simulink model "DC_MOTOR_CONTROL_SIMULACION"  (R2022b)
settings: Solver=ode45  StartTime=0.0  StopTime=100  RelTol=1e-3
values from neighbouring files (symbols this model uses):
  B = 5.076    [dc_motor_control_design.m]
libraries: fod x1
settings Model: Creator=mario  LastModifiedBy=mario
settings SolverCC: ZeroCrossAlgorithm=Adaptive
settings DebuggingCC: IgnoredZcDiagnostic=none

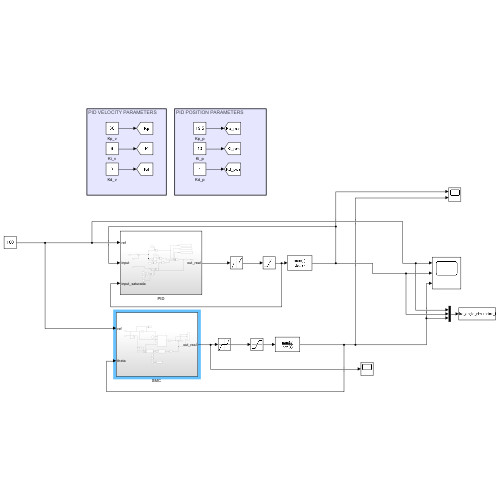
[thumbnail: Simulink's stored preview of the top-level diagram]
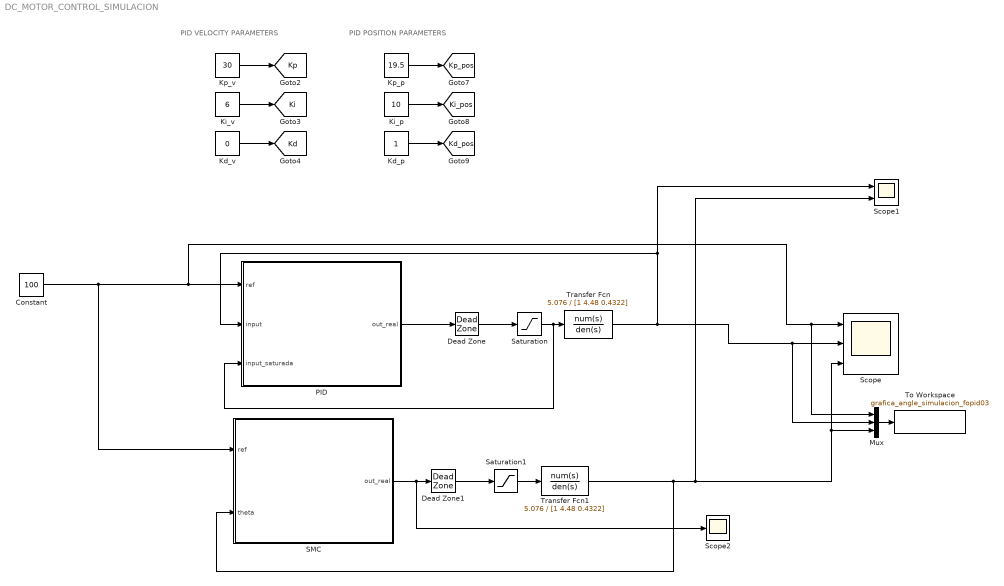
== system DC_MOTOR_CONTROL_SIMULACION ==
  note: PID VELOCITY PARAMETERS
  note: PID POSITION PARAMETERS
  Constant : Constant  Value=100
  Dead Zone : DeadZone  LowerValue=-70  UpperValue=70
  Dead Zone1 : DeadZone  LowerValue=-70  UpperValue=70
  Kd_p : Constant
  Kd_v : Constant  Value=0
  Ki_p : Constant  Value=10
  Ki_v : Constant  Value=6
  Kp_p : Constant  Value=19.5
  Kp_v : Constant  Value=30
  Mux : Mux  Inputs=3
  PID : Subsystem
  "SMC " : Subsystem
  Saturation : Saturate  UpperLimit=255  LowerLimit=-255
  Saturation1 : Saturate  UpperLimit=255  LowerLimit=-255
  Scope : Scope  NumInputPorts=3
  Scope1 : Scope  NumInputPorts=2
  Scope2 : Scope
  To Workspace : ToWorkspace  VariableName=grafica_angle_simulacion_fopid03  SampleTime=0.01
  Transfer Fcn : TransferFcn  Numerator=5.076  Denominator=[1 4.48 0.4322]
  Transfer Fcn1 : TransferFcn  Numerator=5.076  Denominator=[1 4.48 0.4322]
  tag scope: Kd=global, Kd_pos=global, Ki=global, Ki_pos=global, Kp=global, Kp_pos=global
  wires:
  Constant/1 -> "SMC "/1(ref), PID/1(ref), Mux/1, Scope/1
  PID/1(out_real) -> Dead Zone/1
  Dead Zone/1 -> Saturation/1
  Saturation/1 -> PID/3(input_saturada), Transfer Fcn/1
  Transfer Fcn/1 -> PID/2(input), Scope1/1, Mux/2, Scope/2
  "SMC "/1(out_real) -> Scope2/1, Dead Zone1/1
  Saturation1/1 -> Transfer Fcn1/1
  Transfer Fcn1/1 -> "SMC "/2(theta), Scope1/2, Mux/3, Scope/3
  Kp_v/1 -> [Kp]
  Ki_v/1 -> [Ki]
  Kp_p/1 -> [Kp_pos]
  Kd_v/1 -> [Kd]
  Kd_p/1 -> [Kd_pos]
  Ki_p/1 -> [Ki_pos]
  Dead Zone1/1 -> Saturation1/1
  Mux/1 -> To Workspace/1

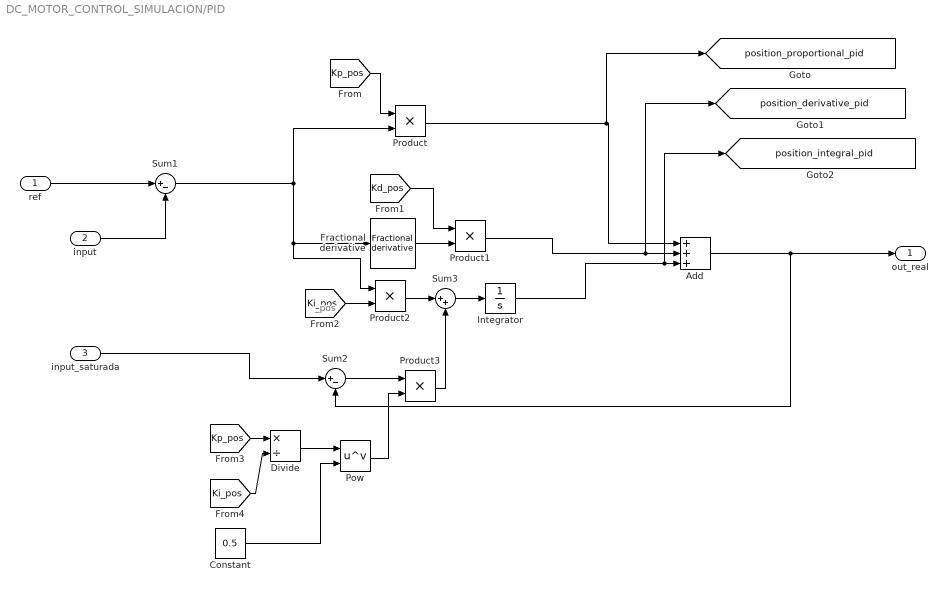
== system DC_MOTOR_CONTROL_SIMULACION/PID ==
  note: _pos
  ref : Inport
  input : Inport  Port=2
  input_saturada : Inport  Port=3
  Add : Sum  Inputs=+++
  Constant : Constant  Value=0.5
  Divide : Product  Inputs=*/
  Fractional derivative : fod/Fractional derivative  gam=1  ww=[0.1; 50]  n=5  nFod=off
      settings: SourceProductName=FOMCON Toolbox
  Integrator : Integrator
  Pow : Math  Operator=pow  SignedPower=on  RndMeth=Zero
  Product{,1..3} (4 alike) : Product
  Sum1 : Sum  Inputs=|+-
  Sum2 : Sum  Inputs=|+-
  Sum3 : Sum  Inputs=|++
  out_real : Outport
  tag scope: position_derivative_pid=global, position_integral_pid=global, position_proportional_pid=global
  wires:
  ref/1 -> Sum1/1
  input/1 -> Sum1/2
  Add/1 -> Sum2/2, out_real/1
  Product/1 -> [position_proportional_pid], Add/1
  Sum1/1 -> Fractional derivative/1, Product2/1, Product/2
  Product1/1 -> Add/2, [position_derivative_pid]
  Product2/1 -> Sum3/1
  Sum3/1 -> Integrator/1
  Sum2/1 -> Product3/1
  Integrator/1 -> [position_integral_pid], Add/3
  input_saturada/1 -> Sum2/1
  Fractional derivative/1 -> Product1/2
  [Kp_pos] -> Product/1
  [Kd_pos] -> Product1/1
  [Ki_pos] -> Product2/2
  [Kp_pos] -> Divide/1
  [Ki_pos] -> Divide/2
  Divide/1 -> Pow/1
  Constant/1 -> Pow/2
  Pow/1 -> Product3/2
  Product3/1 -> Sum3/2

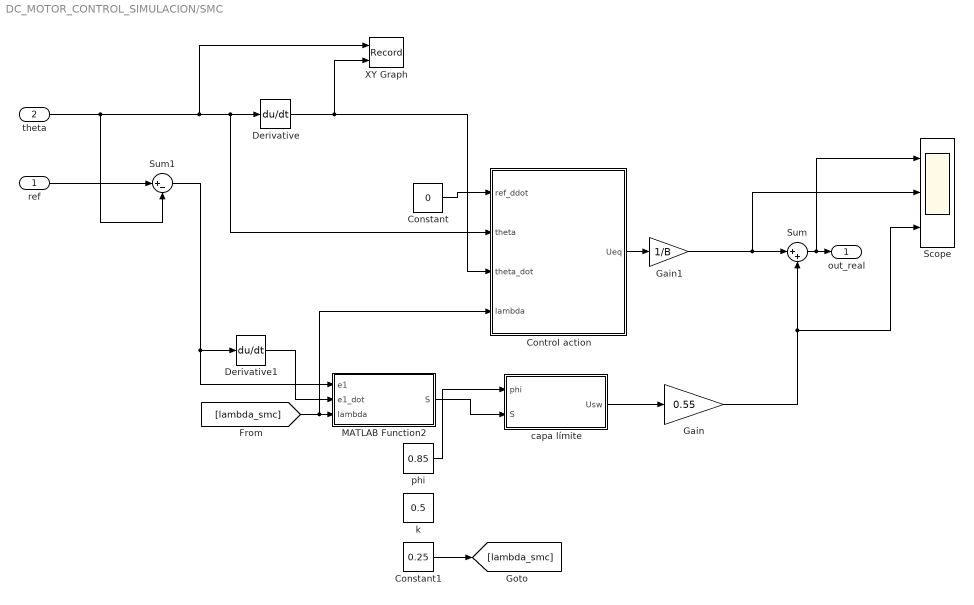
== system DC_MOTOR_CONTROL_SIMULACION/SMC  ==
  ref : Inport
  theta : Inport  Port=2
  Constant : Constant  Value=0
  Constant1 : Constant  Value=0.25
  Control action : MATLAB Function  TreatAsAtomicUnit=on
  Derivative : Derivative
  Derivative1 : Derivative
  Gain : Gain  Gain=0.55
  Gain1 : Gain  Gain=1/B
  MATLAB Function2 : MATLAB Function  TreatAsAtomicUnit=on
  Scope : Scope  NumInputPorts=3
  Sum : Sum  Inputs=|++
  Sum1 : Sum  Inputs=|+-
  XY Graph : Record  FileSettingsInternal="{\"entries\":[{\"content\":{\"excelSettings\":{\"content\":{},\"type\":\"Streamout.ExcelSettings\"}},\"type\":\"Streamout.FileSettingStorage\",\"uuid\":\"\"}],\"packageUris\":[\"http:\\/\\/schema.mathworks.com\\/mf0\\/streamout_blocks\\/R2020a\"],\"version\":\"1.0\"}"  Layout=[1 1]  SignalsInternal="{\"entries\":[{\"content\":{\"signals\":[{\"content\":{\"blockPath\":[],\"channel\":[],\"dimensions\":[1],\"domain\":\"\",\"lineColor\":\"#a2142f\",\"plots\":[1],\"port\":1,\"sid\":[\"\"],\"signalID\":769764,\"signalName\":\"theta\"},\"type\":\"RecordBlkView.Signal\",\"uuid\":\"\"},{\"content\":{\"blockPath\":[],\"channel\":[],\"dimensions\":[1],\"domain\":\"\",\"lineColor\":\"#139fff\",\"plots\":[1],\"port\":2,\"sid\":[\"\"],\"signalID\":769768,\"signalName\":\"Derivative\"},\"type\":\"RecordBlkView.Signal\",\"uuid\":\"\"}]},\"type\":\"RecordBlkView.InputSignals\",\"uuid\":\"\"}],\"packageUris\":[\"http:\\/\\/schema.mathworks.com\\/mf0\\/streamout_blocks\\/R2020a\"],\"version\":\"1.0\"}"  VisualizationBindings="{\"xyplotplugin\":{\"info\":[{\"series\":[{\"bindingParametersList\":[{\"parameter\":\"X-Axis\",\"signalID\":769764,\"signalName\":\"theta\"},{\"parameter\":\"Y-Axis\",\"signalID\":769768,\"signalName\":\"Derivative\"}],\"seriesID\":57437}],\"subplotID\":1}]}}"  CompatibilityTag=XY
  capa límite : MATLAB Function  TreatAsAtomicUnit=on
  k : Constant  Value=0.5
  phi : Constant  Value=0.85
  out_real : Outport
  wires:
  ref/1 -> Sum1/1
  theta/1 -> XY Graph/1, Control action/2(theta), Derivative/1, Sum1/2
  Constant/1 -> Control action/1(ref_ddot)
  Sum1/1 -> Derivative1/1, MATLAB Function2/1(e1)
  Constant1/1 -> [lambda_smc]
  [lambda_smc] -> Control action/4(lambda), MATLAB Function2/3(lambda)
  Sum/1 -> Scope/1, out_real/1
  Control action/1(Ueq) -> Gain1/1
  Gain1/1 -> Scope/2, Sum/1
  capa límite/1(Usw) -> Gain/1
  Derivative/1 -> XY Graph/2, Control action/3(theta_dot)
  Derivative1/1 -> MATLAB Function2/2(e1_dot)
  MATLAB Function2/1(S) -> capa límite/2(S)
  phi/1 -> capa límite/1(phi)
  Gain/1 -> Scope/3, Sum/2

== matlab function DC_MOTOR_CONTROL_SIMULACION/SMC /capa límite ==
  data: Usw output; phi input; S input
function Usw = fcn(phi,S)

if((S/phi)>=1)
    Usw = sign(S/phi);
else
    Usw = S/phi;
end

== matlab function DC_MOTOR_CONTROL_SIMULACION/SMC /Control action ==
  data: Ueq output; ref_ddot input; theta input; theta_dot input; lambda input
function Ueq = fcn(ref_ddot,theta,theta_dot, lambda)

Ueq = (ref_ddot + 0.4322*theta + (4.48-lambda)*theta_dot);

== matlab function DC_MOTOR_CONTROL_SIMULACION/SMC /MATLAB Function2 ==
  data: S output; e1 input; e1_dot input; lambda input
function S = fcn(e1,e1_dot, lambda)

S = lambda*e1 + e1_dot;
